simulink model "springblockdiagram"  (R2024a)
settings: Solver=VariableStepAuto  StartTime=0.0  StopTime=10.0  RelTol=1e-3
undefined symbols (not defined in the file): b, k, m
settings Model: Creator=adithya  LastModifiedBy=adithya

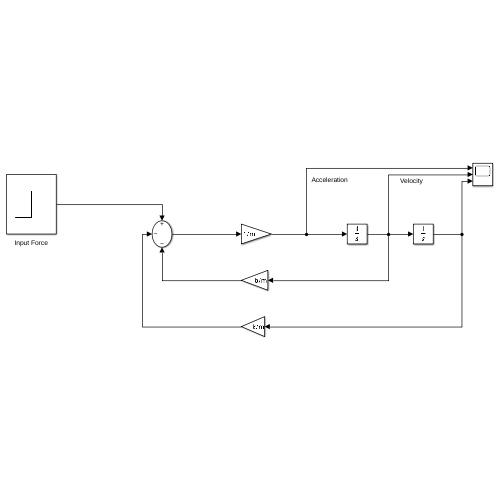
[thumbnail: Simulink's stored preview of the top-level diagram]
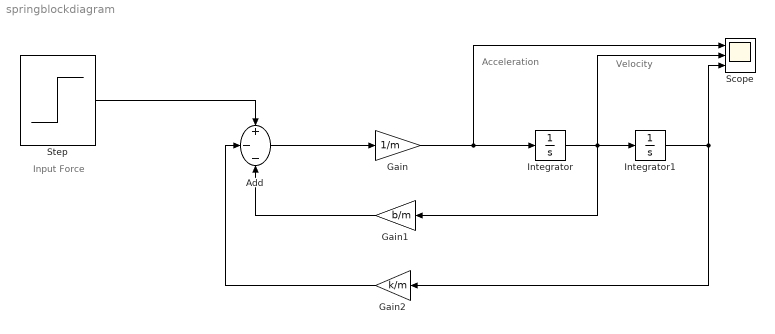
== system springblockdiagram ==
  note: Velocity
  note: Acceleration
  note: Input Force
  Add : Sum  Inputs=+--
  Gain : Gain  Gain=1/m
  Gain1 : Gain  Gain=b/m
  Gain2 : Gain  Gain=k/m
  Integrator : Integrator
  Integrator1 : Integrator
  Scope : Scope  NumInputPorts=3
  Step : Step  SampleTime=0
  wires:
  Step/1 -> Add/1
  Add/1 -> Gain/1
  Gain/1 -> Scope/1, Integrator/1
  Integrator/1 -> Scope/2, Gain1/1, Integrator1/1
  Integrator1/1 -> Gain2/1, Scope/3
  Gain1/1 -> Add/3
  Gain2/1 -> Add/2
